simulink model "Z1"  (R2015b)
settings: Solver=FixedStepAuto  StartTime=0.0  StopTime=10.0  FixedStep=0.001  RelTol=1e-3
settings Model: Creator=Erdal  LastModifiedBy=Erdal

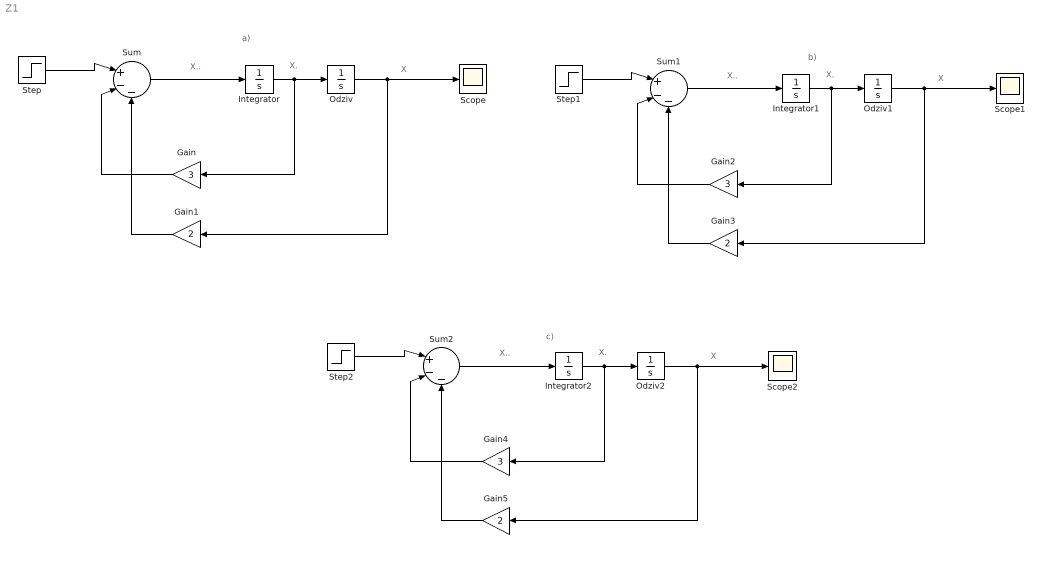
== system Z1 ==
  note: c)
  note: b)
  note: a)
  note: X
  note: X.
  note: X..
  note: X
  note: X.
  note: X..
  note: X
  note: X.
  note: X..
  Gain : Gain  Gain=3
  Gain1 : Gain  Gain=2
  Gain2 : Gain  Gain=3
  Gain3 : Gain  Gain=2
  Gain4 : Gain  Gain=3
  Gain5 : Gain  Gain=2
  Integrator : Integrator
  Integrator1 : Integrator
  Integrator2 : Integrator  InitialCondition=1
  Odziv : Integrator
  Odziv1 : Integrator
  Odziv2 : Integrator  InitialCondition=0.5
  Scope : Scope
  Scope1 : Scope
  Scope2 : Scope
  Step : Step  Time=4  SampleTime=0
  Step1 : Step  Time=4  SampleTime=0
  Step2 : Step  Time=4  SampleTime=0
  Sum : Sum  Inputs=|+--
  Sum1 : Sum  Inputs=|+--
  Sum2 : Sum  Inputs=|+--
  wires:
  Step/1 -> Sum/1
  Sum/1 -> Integrator/1
  Integrator/1 -> Gain/1, Odziv/1
  Odziv/1 -> Gain1/1, Scope/1
  Gain1/1 -> Sum/3
  Gain/1 -> Sum/2
  Step1/1 -> Sum1/1
  Sum1/1 -> Integrator1/1
  Integrator1/1 -> Odziv1/1, Gain2/1
  Odziv1/1 -> Scope1/1, Gain3/1
  Gain3/1 -> Sum1/3
  Gain2/1 -> Sum1/2
  Step2/1 -> Sum2/1
  Sum2/1 -> Integrator2/1
  Integrator2/1 -> Gain4/1, Odziv2/1
  Odziv2/1 -> Gain5/1, Scope2/1
  Gain5/1 -> Sum2/3
  Gain4/1 -> Sum2/2
